simulink model "simulation_02"  (R2022a)
settings: Solver=VariableStepAuto  StartTime=0.0  StopTime=25  RelTol=1e-3
settings Model: Creator=Eshmith  LastModifiedBy=Eshmith

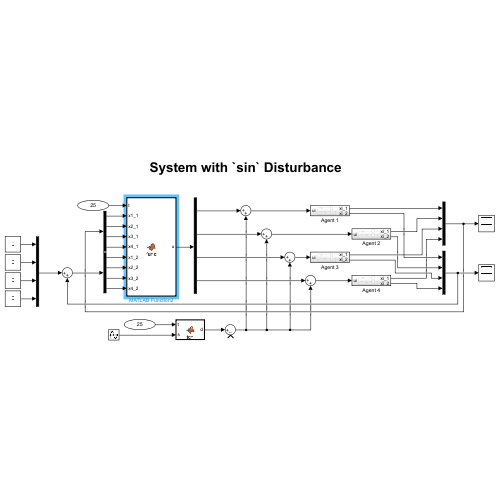
[thumbnail: Simulink's stored preview of the top-level diagram]
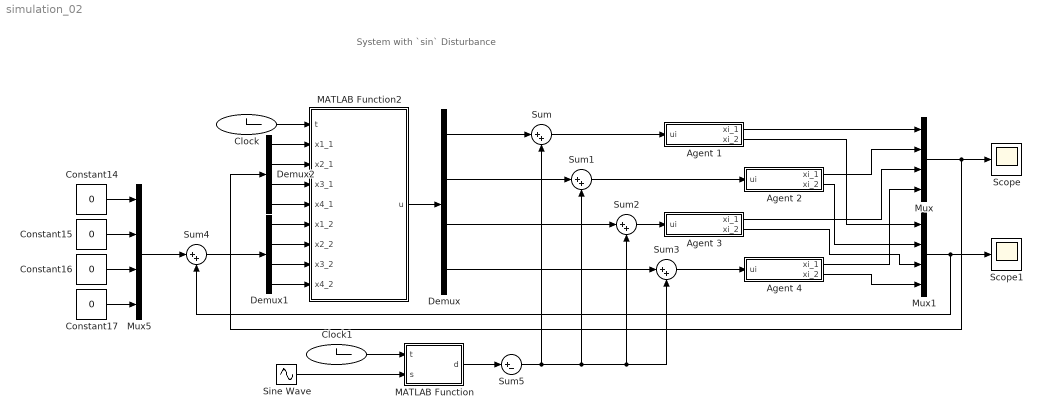
== system simulation_02 ==
  note: System with `sin` Disturbance
  Agent 1 : Subsystem
  Agent 2 : Subsystem
  Agent 3 : Subsystem
  Agent 4 : Subsystem
  Clock : Clock
  Clock1 : Clock
  Constant{14..17} (4 alike) : Constant  Value=0
  Demux : Demux
  Demux1 : Demux
  Demux2 : Demux
  MATLAB Function : MATLAB Function  TreatAsAtomicUnit=on
  MATLAB Function2 : MATLAB Function  TreatAsAtomicUnit=on
  Mux : Mux
  Mux1 : Mux
  Mux5 : Mux
  Scope : Scope
  Scope1 : Scope
  Sine Wave : Sin  SineType=Sample based  Samples=100  SampleTime=0.01
  Sum{,1..4} (5 alike) : Sum  Inputs=|++
  Sum5 : Sum  Inputs=|+-
  wires:
  Clock/1 -> MATLAB Function2/1(t)
  MATLAB Function2/1(u) -> Demux/1
  Demux/1 -> Sum/1
  Demux/2 -> Sum1/1
  Demux/3 -> Sum2/1
  Demux/4 -> Sum3/1
  Sum/1 -> Agent 1/1(ui)
  Sum1/1 -> Agent 2/1(ui)
  Sum2/1 -> Agent 3/1(ui)
  Sum3/1 -> Agent 4/1(ui)
  MATLAB Function/1(d) -> Sum5/1
  Agent 1/1(xi_1) -> Mux/1
  Agent 2/1(xi_1) -> Mux/2
  Agent 3/1(xi_1) -> Mux/3
  Agent 4/1(xi_1) -> Mux/4
  Agent 1/2(xi_2) -> Mux1/1
  Agent 2/2(xi_2) -> Mux1/2
  Agent 3/2(xi_2) -> Mux1/3
  Agent 4/2(xi_2) -> Mux1/4
  Mux1/1 -> Sum4/2, Scope1/1
  Demux1/1 -> MATLAB Function2/6(x1_2)
  Demux1/2 -> MATLAB Function2/7(x2_2)
  Demux1/3 -> MATLAB Function2/8(x3_2)
  Demux1/4 -> MATLAB Function2/9(x4_2)
  Mux/1 -> Scope/1, Demux2/1
  Demux2/1 -> MATLAB Function2/2(x1_1)
  Demux2/2 -> MATLAB Function2/3(x2_1)
  Demux2/3 -> MATLAB Function2/4(x3_1)
  Demux2/4 -> MATLAB Function2/5(x4_1)
  Constant16/1 -> Mux5/3
  Sum4/1 -> Demux1/1
  Mux5/1 -> Sum4/1
  Constant14/1 -> Mux5/1
  Constant15/1 -> Mux5/2
  Constant17/1 -> Mux5/4
  Sum5/1 -> Sum3/2, Sum2/2, Sum1/2, Sum/2
  Sine Wave/1 -> MATLAB Function/2(s)
  Clock1/1 -> MATLAB Function/1(t)

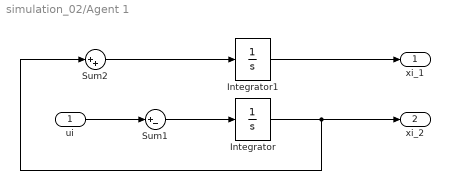
== system simulation_02/Agent 1 ==
  ui : Inport
  Integrator : Integrator  InitialCondition=-0.2
  Integrator1 : Integrator  InitialCondition=5
  Sum1 : Sum  Inputs=|+-
  Sum2 : Sum  Inputs=|++
  xi_1 : Outport
  xi_2 : Outport  Port=2
  wires:
  Sum1/1 -> Integrator/1
  ui/1 -> Sum1/1
  Integrator/1 -> Sum2/1, xi_2/1
  Integrator1/1 -> xi_1/1
  Sum2/1 -> Integrator1/1

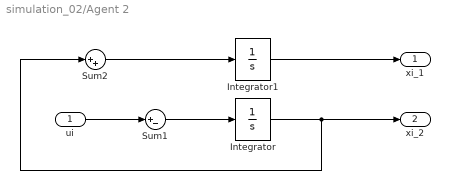
== system simulation_02/Agent 2 ==
  ui : Inport
  Integrator : Integrator  InitialCondition=0.1
  Integrator1 : Integrator  InitialCondition=2
  Sum1 : Sum  Inputs=|+-
  Sum2 : Sum  Inputs=|++
  xi_1 : Outport
  xi_2 : Outport  Port=2
  wires:
  Sum1/1 -> Integrator/1
  ui/1 -> Sum1/1
  Integrator/1 -> Sum2/1, xi_2/1
  Integrator1/1 -> xi_1/1
  Sum2/1 -> Integrator1/1

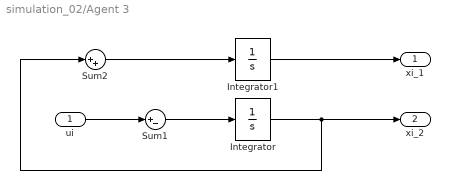
== system simulation_02/Agent 3 ==
  ui : Inport
  Integrator : Integrator  InitialCondition=0.1
  Integrator1 : Integrator  InitialCondition=2
  Sum1 : Sum  Inputs=|+-
  Sum2 : Sum  Inputs=|++
  xi_1 : Outport
  xi_2 : Outport  Port=2
  wires:
  Sum1/1 -> Integrator/1
  ui/1 -> Sum1/1
  Integrator/1 -> Sum2/1, xi_2/1
  Integrator1/1 -> xi_1/1
  Sum2/1 -> Integrator1/1

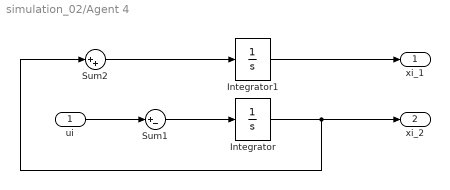
== system simulation_02/Agent 4 ==
  ui : Inport
  Integrator : Integrator  InitialCondition=2
  Integrator1 : Integrator
  Sum1 : Sum  Inputs=|+-
  Sum2 : Sum  Inputs=|++
  xi_1 : Outport
  xi_2 : Outport  Port=2
  wires:
  Sum1/1 -> Integrator/1
  ui/1 -> Sum1/1
  Integrator/1 -> Sum2/1, xi_2/1
  Integrator1/1 -> xi_1/1
  Sum2/1 -> Integrator1/1

== matlab function simulation_02/MATLAB Function ==
  data: t input; d output; s input
function d = fcn(t, s)

if t > 5 && t < 8
    d = s;
else
    d = 0;
end

== matlab function simulation_02/MATLAB Function2 ==
  data: t input; x1_1 input; u output; x2_1 input; x3_1 input; x4_1 input; x1_2 input; x2_2 input; x3_2 input; x4_2 input
function u = func(t, x1_1, x2_1, x3_1, x4_1, x1_2, x2_2, x3_2, x4_2)

states_1 = [x1_1, x2_1, x3_1, x4_1]';
states_2 = [x1_2, x2_2, x3_2, x4_2]';

L = [1.6   0  -0.9  -0.7;
     0     1  -1     0;
    -0.9  -1   1.9   0;
    -0.7   0   0     0.7;
    ];

n = 4;
D = 0.4;
c1 = 2;
c2 = 2.3;
epsilons = [0.02;0.02;0.02;0.02];

eigL = round(eig(L)*10000)/10000;

lambdaMax = max(eigL);

eigs = sort(eigL);
lambdaMin = eigs(2);

S = L*(L*states_2 + c2*L*states_1 + c1*L*states_1*t);

Ebar = max(abs(c1*L*states_1 + c2*L*states_2));

lower_hi = (Ebar + epsilons + sqrt(n)*D*lambdaMax)*sqrt(n)/lambdaMin;

u = real(-lower_hi.*sign(S));

end
